simulink model "EVBatt_WirelessCharging"  (R2020a)
settings: Solver=VariableStepAuto  StartTime=0.0  StopTime=0.5  RelTol=1e-3
undefined symbols (not defined in the file or in its folder): Ion, Lithium
libraries: powerlib x30, electricdrivelib x1
settings Model: Creator=HP  LastModifiedBy=HP
settings SolverCC: ZeroCrossAlgorithm=Adaptive
settings DebuggingCC: IgnoredZcDiagnostic=none

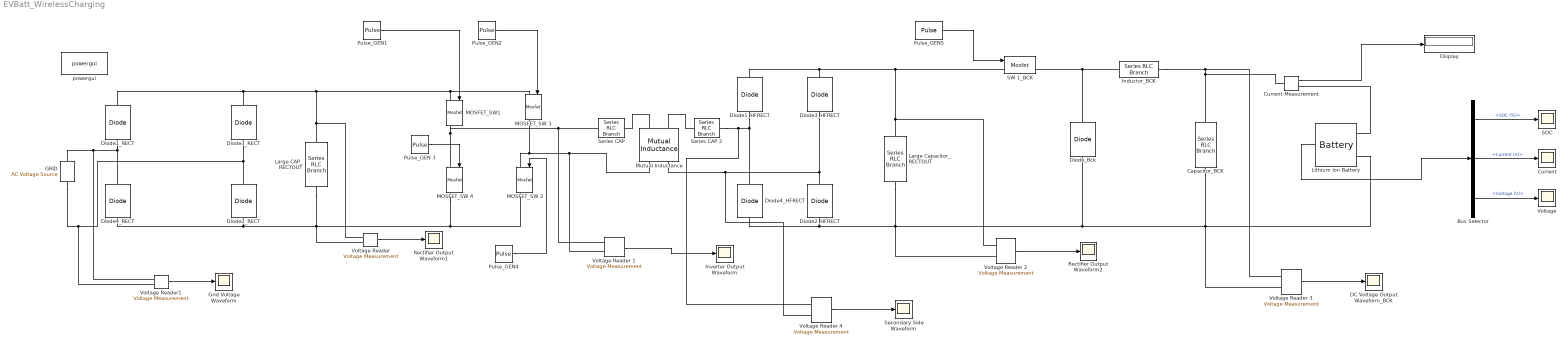
== system EVBatt_WirelessCharging ==
  Bus Selector : BusSelector  OutputSignals=SOC (%),Current (A),Voltage (V)
  Capacitor_BCK : powerlib/Elements/Series RLC Branch  LConnTagsString=__new0  RConnTagsString=__new0  BranchType=C  Resistance=1  Inductance=1e-3  SetiL0=off  InitialCurrent=0  Capacitance=100e-6  Setx0=off  InitialVoltage=0  Measurements=None
  Current : Scope
  Current Measurement : powerlib/Measurements/Current Measurement  PhasorSimulation=off  OutputType=Complex  PSBequivalent=0
  DC Voltage Output Waveform_BCK : Scope
  Diode1_HFRECT : powerlib/Power Electronics/Diode  Ron=0.001  Lon=0  Vf=0.8  IC=0  UseSnubber=0  Rs=500  Cs=250e-9  Measurements=off
  Diode1_RECT : powerlib/Power Electronics/Diode  Ron=0.001  Lon=0  Vf=0.8  IC=0  UseSnubber=0  Rs=500  Cs=250e-9  Measurements=off
  Diode2_HFRECT : powerlib/Power Electronics/Diode  Ron=0.001  Lon=0  Vf=0.8  IC=0  UseSnubber=0  Rs=500  Cs=250e-9  Measurements=off
  Diode2_RECT : powerlib/Power Electronics/Diode  Ron=0.001  Lon=0  Vf=0.8  IC=0  UseSnubber=0  Rs=500  Cs=250e-9  Measurements=off
  Diode3_HFRECT : powerlib/Power Electronics/Diode  Ron=0.001  Lon=0  Vf=0.8  IC=0  UseSnubber=0  Rs=500  Cs=250e-9  Measurements=off
  Diode3_RECT : powerlib/Power Electronics/Diode  Ron=0.001  Lon=0  Vf=0.8  IC=0  UseSnubber=0  Rs=500  Cs=250e-9  Measurements=off
  Diode4_HFRECT : powerlib/Power Electronics/Diode  Ron=0.001  Lon=0  Vf=0.8  IC=0  UseSnubber=0  Rs=500  Cs=250e-9  Measurements=off
  Diode4_RECT : powerlib/Power Electronics/Diode  Ron=0.001  Lon=0  Vf=0.8  IC=0  UseSnubber=0  Rs=500  Cs=250e-9  Measurements=off
  Diode_Bck : powerlib/Power Electronics/Diode  Ron=0.001  Lon=0  Vf=0.8  IC=0  UseSnubber=0  Rs=500  Cs=250e-9  Measurements=off
  Display : Display
  GRID : powerlib/Electrical Sources/AC Voltage Source  Amplitude=240  Phase=0  Frequency=50  SampleTime=0  Measurements=None  BusType=swing  Pref=10e3  Qref=0  Qmin=-inf  Qmax=+inf
  Grid Voltage Waveform : Scope
  Inductor_BCK : powerlib/Elements/Series RLC Branch  LConnTagsString=__new0  RConnTagsString=__new0  BranchType=L  Resistance=1  Inductance=750e-3  SetiL0=off  InitialCurrent=0  Capacitance=1000e-6  Setx0=off  InitialVoltage=0  Measurements=None
  Inverter Output Waveform : Scope
  Large CAP_RECTOUT : powerlib/Elements/Series RLC Branch  LConnTagsString=__new0  RConnTagsString=__new0  BranchType=C  Resistance=1  Inductance=1e-3  SetiL0=off  InitialCurrent=0  Capacitance=70000e-6  Setx0=off  InitialVoltage=0  Measurements=None
  Large Capacitor_RECTOUT : powerlib/Elements/Series RLC Branch  LConnTagsString=__new0  RConnTagsString=__new0  BranchType=C  Resistance=1  Inductance=1e-3  SetiL0=off  InitialCurrent=0  Capacitance=1000e-6  Setx0=off  InitialVoltage=0  Measurements=None
  Lithium Ion Battery : electricdrivelib/Extra Sources/Battery  BatType=Lithium-Ion  ShowTempParam=off  ThermalPreset=no  ShowAgeParam=off  NomV=3  NomQ=2.2  SOC=80  Batt_Tr=30  PresetModel=on  MaxQ=2.2  MinV=2.25  FullV=3.492  Dis_rate=0.95652  R=0.013636  Normal_OP=1.9896  expZone="[3.2412     0.10809]"  current=[6.5 13 32.5]  Units=Time  Tci=20  NomT=20  T2=-30  MaxQ2=4.8  FullV2=7.1  Normal_OP2=5.655  expZone2="[6.58           1]"  Rca=0.6  ti=2000  Dp=0  Neq0=0  Tsim=1e6  Ta1=25  Qeol=5.4*0.9  Reol=0.013333*1.2  Char_age=[2.3478, 3]  Dis_age=[2.3478, 10]  N1=1500  N2=10500  N3=1000  N4=1400  Ta2=45  N5=950
  MOSFET_SW 2 : powerlib/Power Electronics/Mosfet  Ron=0.1  Lon=0  Rd=0.01  Vfd=0  IC=0  Rs=1e5  Cs=inf  Measurements=on
  MOSFET_SW 3 : powerlib/Power Electronics/Mosfet  Ron=0.1  Lon=0  Rd=0.01  Vfd=0  IC=0  Rs=1e5  Cs=inf  Measurements=on
  MOSFET_SW 4 : powerlib/Power Electronics/Mosfet  Ron=0.1  Lon=0  Rd=0.01  Vfd=0  IC=0  Rs=1e5  Cs=inf  Measurements=on
  MOSFET_SW1 : powerlib/Power Electronics/Mosfet  Ron=0.1  Lon=0  Rd=0.01  Vfd=0  IC=0  Rs=1e5  Cs=inf  Measurements=on
  Mutual Inductance : powerlib/Elements/Mutual Inductance  LConnTagsString=a|b  RConnTagsString=A|B  TypeOfMutual=Two or three windings with equal mutual terms  NumberOfWindings=3  SelfImpedance1=[0.0714 73.43e-06]  SelfImpedance2=[0.0714 73.43e-06]  ThreeWindings=off  SelfImpedance3=[ 1.1 1.1e-03]  MutualImpedance=[0.142 1.46e-05]  InductanceMatrix="[1.0 0.9  0.9 ;  0.9 1.0  0.9;  0.9 0.9 1.0 ] * 1e-3"  ResistanceMatrix="[1.0 0.9  0.9 ;  0.9 1.0  0.9;  0.9 0.9 1.0 ]"  Measurements=None
      settings: AttributesFormatString=\n  SourceProductBaseCode=PS
  Pulse_GEN 3 : DiscretePulseGenerator  PulseType=Time based  Period=0.02  PulseWidth=50  PhaseDelay=0.01
  Pulse_GEN1 : DiscretePulseGenerator  PulseType=Time based  Period=0.02  PulseWidth=50
  Pulse_GEN2 : DiscretePulseGenerator  PulseType=Time based  Period=0.02  PulseWidth=50  PhaseDelay=0.01
  Pulse_GEN4 : DiscretePulseGenerator  PulseType=Time based  Period=0.02  PulseWidth=50
  Pulse_GEN5 : DiscretePulseGenerator  PulseType=Time based  Period=0.02  PulseWidth=50
  Rectifier Output Waveform1 : Scope
  Rectifier Output Waveform2 : Scope
  SOC : Scope
  SW 1_BCK : powerlib/Power Electronics/Mosfet  Ron=0.1  Lon=0  Rd=0.01  Vfd=0  IC=0  Rs=1e5  Cs=inf  Measurements=on
  Secondary Side Waveform : Scope
  Series CAP : powerlib/Elements/Series RLC Branch  LConnTagsString=__new0  RConnTagsString=__new0  BranchType=C  Resistance=1  Inductance=1e-3  SetiL0=off  InitialCurrent=0  Capacitance=0.2e-6  Setx0=off  InitialVoltage=0  Measurements=None
  Series CAP 2 : powerlib/Elements/Series RLC Branch  LConnTagsString=__new0  RConnTagsString=__new0  BranchType=C  Resistance=1  Inductance=1e-3  SetiL0=off  InitialCurrent=0  Capacitance=0.2e-6  Setx0=off  InitialVoltage=0  Measurements=None
  Voltage : Scope
  Voltage Reader : powerlib/Measurements/Voltage Measurement  PhasorSimulation=off  OutputType=Complex  PSBequivalent=0
  Voltage Reader {1..4} (4 alike) : powerlib/Measurements/Voltage Measurement  PhasorSimulation=off  OutputType=Complex  PSBequivalent=0
  Voltage Reader1 : powerlib/Measurements/Voltage Measurement  PhasorSimulation=off  OutputType=Complex  PSBequivalent=0
  powergui : powerlib/powergui  Priority=1  SimulationMode=Continuous  SampleTime=50e-6  frequency=60  Iterations=50  frequencyindice=0  Pbase=100e6  ErrMax=1e-4  UnitsV=kV  UnitsW=MW  buscounter=0  FunctionMessages=off  echomessages=off  EnableUseOfTLC=off  CurrentSourceSwitches=off  DisableSnubberDevices=off  DisableRonSwitches=off  DisableVfSwitches=off  DisplayEquations=off  AutomaticDiscreteSolvers=off  SolverType=Tustin/Backward Euler (TBE)  Interpol=off  ExternalGateDelay=off  methode=off  Ts=100  x0status=blocks  SPID=on  SwTol=0  HookPort=off  NonlinearTolerance=1e-4  nMaxIteration=100  ContinueOnMaxIteration=off  RestoreLinks=warning  ResistiveCurrentMeasurement=off  Frange=[0:2:500]  Ylog=off  Xlog=on  ShowGrid=off  save=off  variable=ZData  structure=0  ZoomFFT=off  StartTime=0.0  cycles=1  DisplayStyle=1  fundamental=60  FreqAxis=off  MaxFrequency=1000  frequencyindicesteady=1  RmsSteady=1  display=off
  wires:
  Voltage Reader/1 -> Rectifier Output Waveform1/1
  Pulse_GEN1/1 -> MOSFET_SW1/1
  Pulse_GEN4/1 -> MOSFET_SW 2/1
  Pulse_GEN 3/1 -> MOSFET_SW 4/1
  Pulse_GEN2/1 -> MOSFET_SW 3/1
  Voltage Reader 2/1 -> Rectifier Output Waveform2/1
  Pulse_GEN5/1 -> SW 1_BCK/1
  Lithium Ion Battery/1 -> Bus Selector/1
  Bus Selector/1 -> SOC/1  "<SOC (%)>"
  Bus Selector/2 -> Current/1  "<Current (A)>"
  Bus Selector/3 -> Voltage/1  "<Voltage (V)>"
  Voltage Reader 1/1 -> Inverter Output Waveform/1
  Voltage Reader 3/1 -> DC Voltage Output Waveform_BCK/1
  Current Measurement/1 -> Display/1
  Voltage Reader 4/1 -> Secondary Side Waveform/1
  Voltage Reader1/1 -> Grid Voltage Waveform/1
  connections:
  Diode1_RECT/LConn1 -- GRID/RConn1 -- Voltage Reader1/LConn1 -- Diode4_RECT/RConn1
  Diode3_RECT/LConn1 -- Voltage Reader1/LConn2 -- GRID/LConn1 -- Diode2_RECT/RConn1
  MOSFET_SW1/RConn1 -- Series CAP/LConn1 -- Voltage Reader 1/LConn1 -- MOSFET_SW 4/LConn1
  MOSFET_SW 3/RConn1 -- Mutual Inductance/LConn1 -- Voltage Reader 1/LConn2 -- MOSFET_SW 2/LConn1
  Diode1_RECT/RConn1 -- Large CAP_RECTOUT/RConn1 -- Voltage Reader/LConn1 -- MOSFET_SW 3/LConn1 -- MOSFET_SW1/LConn1 -- Diode3_RECT/RConn1
  Diode4_RECT/LConn1 -- MOSFET_SW 4/RConn1 -- MOSFET_SW 2/RConn1 -- Large CAP_RECTOUT/LConn1 -- Voltage Reader/LConn2 -- Diode2_RECT/LConn1
  Mutual Inductance/RConn1 -- Series CAP/RConn1
  Series CAP 2/LConn1 -- Mutual Inductance/RConn2
  Diode1_HFRECT/RConn1 -- Voltage Reader 2/LConn1 -- Large Capacitor_RECTOUT/RConn1 -- SW 1_BCK/LConn1 -- Diode3_HFRECT/RConn1
  Diode4_HFRECT/LConn1 -- Voltage Reader 2/LConn2 -- Capacitor_BCK/RConn1 -- Lithium Ion Battery/LConn2 -- Voltage Reader 3/LConn2 -- Diode_Bck/LConn1 -- Large Capacitor_RECTOUT/LConn1 -- Diode2_HFRECT/LConn1
  Diode1_HFRECT/LConn1 -- Voltage Reader 4/LConn1 -- Series CAP 2/RConn1 -- Diode4_HFRECT/RConn1
  Diode3_HFRECT/LConn1 -- Voltage Reader 4/LConn2 -- Mutual Inductance/LConn2 -- Diode2_HFRECT/RConn1
  Diode_Bck/RConn1 -- Inductor_BCK/LConn1 -- SW 1_BCK/RConn1
  Inductor_BCK/RConn1 -- Capacitor_BCK/LConn1 -- Current Measurement/LConn1 -- Voltage Reader 3/LConn1
  Lithium Ion Battery/LConn1 -- Current Measurement/RConn1
